simulink library "Qerror"  (R2014b)
settings: Solver=VariableStepAuto  StartTime=0.0  StopTime=10.0  RelTol=1e-3
undefined symbols (not defined in the file): ConfParam
libraries: Qprod x1
settings Model: Creator=y.akisheva  LastModifiedBy=Hp
settings DataIOCC: SaveFormat=Dataset
settings OptimizationCC: UseDivisionForNetSlopeComputation=off  SimCompilerOptimization=off
settings DebuggingCC: SolverPrmCheckMsg=none  FrameProcessingCompatibilityMsg=error  AllowSymbolicDim=off
settings HardwareCC: ProdBitPerPointer=64  ProdLargestAtomicFloat=Float  ProdIntDivRoundTo=Zero  ProdEndianess=LittleEndian  ProdWordSize=64  ProdHWDeviceType=Intel->x86-64 (Windows64)
settings RTWCC: RTWCompilerOptimization=off
settings GRTTargetCC: GeneratePreprocessorConditionals=Use local settings
settings ConfigComp: CovMetricSettings=dw  CovHtmlReporting=on  CovSaveCumulativeToWorkspaceVar=on  CovSaveSingleToWorkspaceVar=on  CovExternalEMLEnable=off

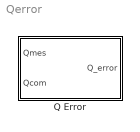
== system Qerror ==
  Q Error : Subsystem

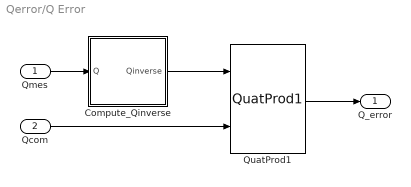
== system Qerror/Q Error ==
  Qmes : Inport
  Qcom : Inport  Port=2
  Compute_Qinverse : Subsystem
  QuatProd1 : Qprod/QuatProd1
  Q_error : Outport
  wires:
  QuatProd1/1 -> Q_error/1
  Qcom/1 -> QuatProd1/2
  Compute_Qinverse/1(Qinverse) -> QuatProd1/1
  Qmes/1 -> Compute_Qinverse/1(Q)

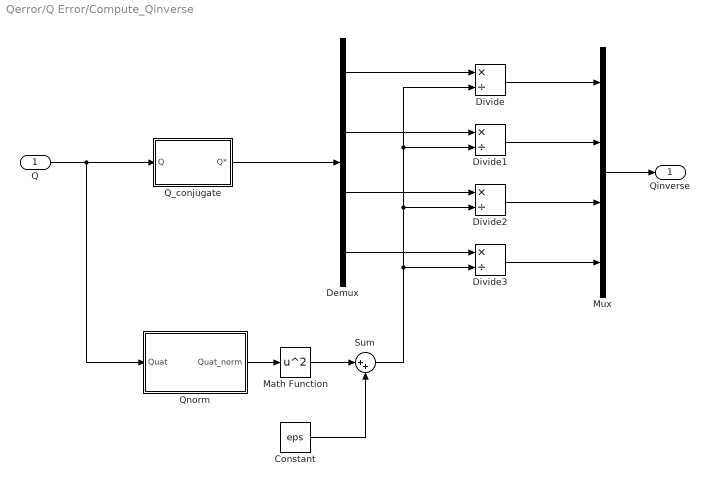
== system Qerror/Q Error/Compute_Qinverse ==
  Q : Inport
  Constant : Constant  Value=eps  SampleTime=1/ConfParam.confES.frequency
  Demux : Demux
  Divide{,1..3} (4 alike) : Product  Inputs=*/
  Math Function : Math  Operator=square  SaturateOnIntegerOverflow=on
  Mux : Mux
  Q_conjugate : Subsystem
  Qnorm : Subsystem
  Sum : Sum  Inputs=|++
  Qinverse : Outport
  wires:
  Constant/1 -> Sum/2
  Math Function/1 -> Sum/1
  Sum/1 -> Divide/2, Divide1/2, Divide2/2, Divide3/2
  Mux/1 -> Qinverse/1
  Demux/2 -> Divide1/1
  Divide2/1 -> Mux/3
  Q_conjugate/1(Q*) -> Demux/1
  Divide/1 -> Mux/1
  Divide1/1 -> Mux/2
  Divide3/1 -> Mux/4
  Q/1 -> Q_conjugate/1(Q), Qnorm/1(Quat)
  Demux/4 -> Divide3/1
  Qnorm/1(Quat_norm) -> Math Function/1
  Demux/1 -> Divide/1
  Demux/3 -> Divide2/1

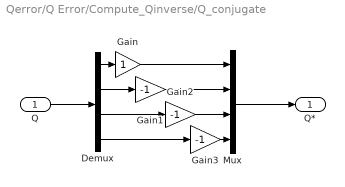
== system Qerror/Q Error/Compute_Qinverse/Q_conjugate ==
  Q : Inport
  Demux : Demux
  Gain : Gain
  Gain1 : Gain  Gain=-1
  Gain2 : Gain  Gain=-1
  Gain3 : Gain  Gain=-1
  Mux : Mux
  Q* : Outport
  wires:
  Gain3/1 -> Mux/4
  Q/1 -> Demux/1
  Gain2/1 -> Mux/3
  Demux/2 -> Gain1/1
  Demux/3 -> Gain2/1
  Gain1/1 -> Mux/2
  Demux/4 -> Gain3/1
  Mux/1 -> Q*/1
  Gain/1 -> Mux/1
  Demux/1 -> Gain/1

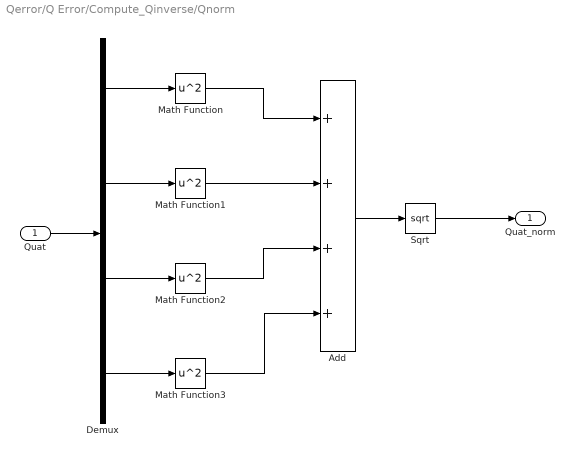
== system Qerror/Q Error/Compute_Qinverse/Qnorm ==
  Quat : Inport
  Add : Sum  Inputs=++++
  Demux : Demux
  Math Function{,1..3} (4 alike) : Math  Operator=square  SaturateOnIntegerOverflow=on
  Sqrt : Sqrt  SaturateOnIntegerOverflow=on
  Quat_norm : Outport
  wires:
  Quat/1 -> Demux/1
  Demux/2 -> Math Function1/1
  Sqrt/1 -> Quat_norm/1
  Demux/4 -> Math Function3/1
  Demux/1 -> Math Function/1
  Demux/3 -> Math Function2/1
  Math Function1/1 -> Add/2
  Math Function3/1 -> Add/4
  Add/1 -> Sqrt/1
  Math Function/1 -> Add/1
  Math Function2/1 -> Add/3
